simulink model "HP_LP_filter"  (R2021b)
settings: Solver=ode1  StartTime=0.0  StopTime=1  FixedStep=0.01  RelTol=1e-3
settings Model: ExtModeTrigDuration=2  Creator=ASUS  LastModifiedBy=ASUS
settings OptimizationCC: DefaultParameterBehavior=Inlined  EnhancedBackFolding=on  PassReuseOutputArgsAs=Individual arguments  ZeroExternalMemoryAtStartup=off  ZeroInternalMemoryAtStartup=off  MaxStackSize=64  OptimizeBlockOrder=speed  DifferentSizesBufferReuse=on  OptimizationCustomize=off  EfficientTunableParamExpr=on
settings DebuggingCC: ParameterTunabilityLossMsg=error
settings HardwareCC: ProdBitPerInt=16  ProdBitPerPointer=16  ProdBitPerSizeT=16  ProdBitPerPtrDiffT=16  ProdLargestAtomicFloat=None  ProdWordSize=8  ProdHWDeviceType=Atmel->AVR
settings SFSimCC: MATLABDynamicMemAlloc=off
settings RTWCC: Description=Embedded Coder  SystemTargetFile=ert.tlc  TemplateMakefile=ert_default_tmf  Toolchain=Arduino AVR  BuildConfiguration=Faster Runs
settings CodeAppCC: ForceParamTrailComments=on  IgnoreCustomStorageClasses=off  OperatorAnnotations=on  SimulinkDataObjDesc=on  SFDataObjDesc=on  InsertBlockDesc=on
settings ERTTargetCC: SupportContinuousTime=on  ExtModeTransport=3  ExtModeStaticAlloc=on  ExtModeStaticAllocSize=2048  ExtModeMexFile=ext_xcp  ExtModeIntrfLevel=Level2 - Open  ERTCustomFileTemplate=example_file_process.tlc

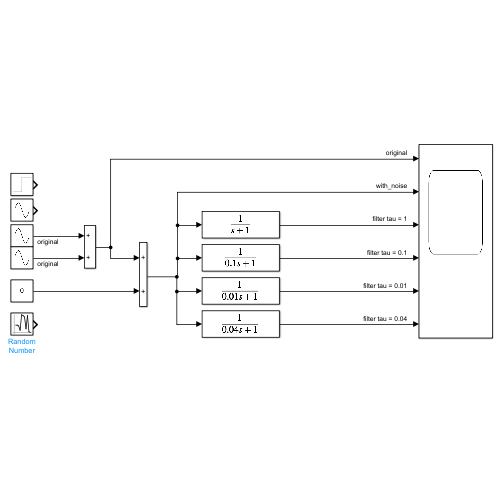
[thumbnail: Simulink's stored preview of the top-level diagram]
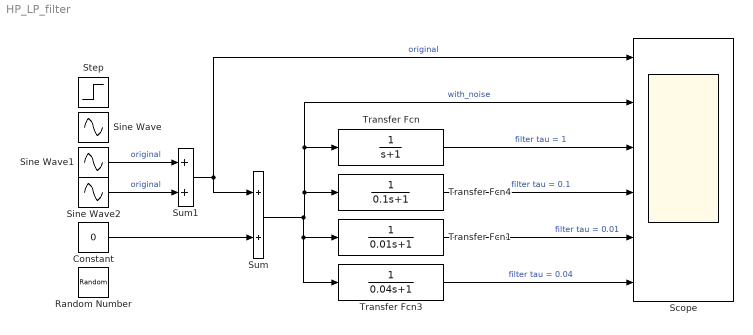
== system HP_LP_filter ==
  Constant : Constant  Value=0
  Random Number : RandomNumber  Variance=0.1  SampleTime=0.01
  Scope : Scope  NumInputPorts=6
  Sine Wave : Sin  Amplitude=5  SampleTime=0
  Sine Wave1 : Sin  Amplitude=5  Frequency=2*pi  SampleTime=0
  Sine Wave2 : Sin  Amplitude=0.1  Frequency=100*pi  SampleTime=0
  Step : Step  SampleTime=0
  Sum : Sum
  Sum1 : Sum
  Transfer Fcn : TransferFcn  Denominator=[1 1]
  Transfer Fcn1 : TransferFcn  Denominator=[0.01 1]
  Transfer Fcn3 : TransferFcn  Denominator=[0.04 1]
  Transfer Fcn4 : TransferFcn  Denominator=[0.1 1]
  wires:
  Sum1/1 -> Sum/1, Scope/1  "original"
  Transfer Fcn/1 -> Scope/3  "filter tau = 1"
  Constant/1 -> Sum/2
  Sum/1 -> Transfer Fcn1/1, Transfer Fcn3/1, Transfer Fcn4/1, Scope/2, Transfer Fcn/1  "with_noise"
  Transfer Fcn3/1 -> Scope/6  "filter tau = 0.04"
  Transfer Fcn1/1 -> Scope/5  "filter tau = 0.01"
  Transfer Fcn4/1 -> Scope/4  "filter tau = 0.1"
  Sine Wave2/1 -> Sum1/2  "original"
  Sine Wave1/1 -> Sum1/1  "original"
